simulink model "ep4_2"  (R2018a)
settings: Solver=FixedStepAuto  StartTime=0.0  StopTime=50  RelTol=1e-3
settings Model: Creator=zheny  LastModifiedBy=zheny

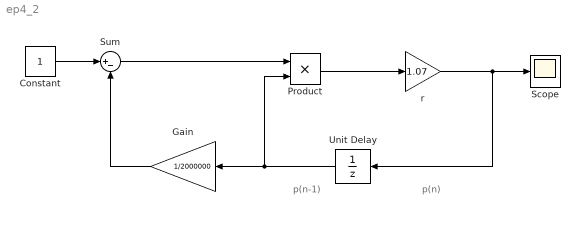
== system ep4_2 ==
  note: p(n)
  note: p(n-1)
  Constant : Constant
  Gain : Gain  Gain=1/2000000
  Product : Product
  Scope : Scope
  Sum : Sum  Inputs=|+-
  Unit Delay : UnitDelay  InitialCondition=500000  SampleTime=-1
  r : Gain  Gain=1.07
  wires:
  Constant/1 -> Sum/1
  r/1 -> Unit Delay/1, Scope/1
  Product/1 -> r/1
  Unit Delay/1 -> Product/2, Gain/1
  Gain/1 -> Sum/2
  Sum/1 -> Product/1
